simulink library "INT_CoME_ShutOff"  (R2016b)
settings: Solver=VariableStepAuto  StartTime=0.0  StopTime=10.0  RelTol=1e-3
settings Model: Creator=Administrator  LastModifiedBy=Administrator

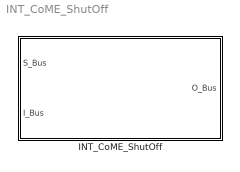
== system INT_CoME_ShutOff ==
  INT_CoME_ShutOff : Subsystem

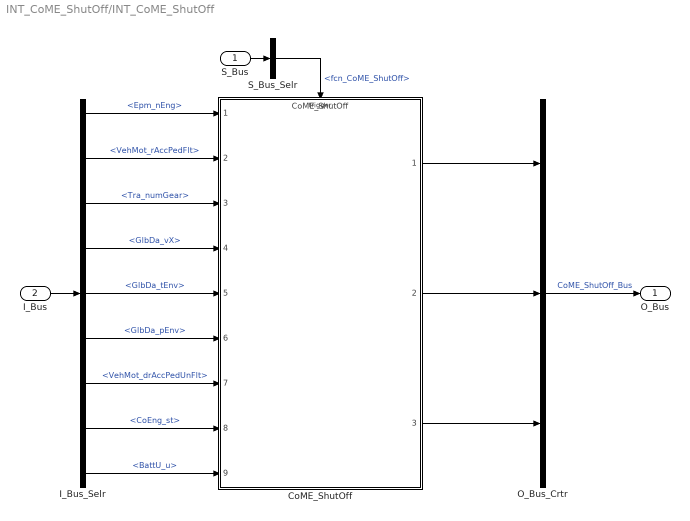
== system INT_CoME_ShutOff/INT_CoME_ShutOff ==
  S_Bus : Inport
  I_Bus : Inport  Port=2
  CoME_ShutOff : ModelReference  ModelNameDialog=CoME_ShutOff  SimulationMode=Normal  ModelReferenceVersion=1.22  TriggerPortName=function  TriggerPortTriggerType=function-call  TriggerPortStatesWhenEnabling=held
  I_Bus_Selr : BusSelector  OutputSignals=Epm_nEng,VehMot_rAccPedFlt,Tra_numGear,GlbDa_vX,GlbDa_tEnv,GlbDa_pEnv,VehMot_drAccPedUnFlt,CoEng_st,BattU_u
  O_Bus_Crtr : BusCreator  Inputs=3
  S_Bus_Selr : BusSelector  OutputSignals=fcn_CoME_ShutOff
  O_Bus : Outport
  wires:
  S_Bus_Selr/1 -> CoME_ShutOff/Trigger  "<fcn_CoME_ShutOff>"
  S_Bus/1 -> S_Bus_Selr/1
  I_Bus/1 -> I_Bus_Selr/1
  I_Bus_Selr/1 -> CoME_ShutOff/1  "<Epm_nEng>"
  I_Bus_Selr/2 -> CoME_ShutOff/2  "<VehMot_rAccPedFlt>"
  I_Bus_Selr/3 -> CoME_ShutOff/3  "<Tra_numGear>"
  I_Bus_Selr/4 -> CoME_ShutOff/4  "<GlbDa_vX>"
  I_Bus_Selr/5 -> CoME_ShutOff/5  "<GlbDa_tEnv>"
  I_Bus_Selr/6 -> CoME_ShutOff/6  "<GlbDa_pEnv>"
  I_Bus_Selr/7 -> CoME_ShutOff/7  "<VehMot_drAccPedUnFlt>"
  I_Bus_Selr/8 -> CoME_ShutOff/8  "<CoEng_st>"
  I_Bus_Selr/9 -> CoME_ShutOff/9  "<BattU_u>"
  O_Bus_Crtr/1 -> O_Bus/1  "CoME_ShutOff_Bus"
  CoME_ShutOff/1 -> O_Bus_Crtr/1
  CoME_ShutOff/2 -> O_Bus_Crtr/2
  CoME_ShutOff/3 -> O_Bus_Crtr/3
